simulink model "main_simplify"  (R2022a)
settings: Solver=ode4  StartTime=0.0  StopTime=1000  FixedStep=0.1  RelTol=1e-3
undefined symbols (not defined in the file): X, Y, Z
libraries: nesl_utility x28, sm_lib x9, sharedtransform x1
(part 1 of 2)
settings Model: Creator=sakur  LastModifiedBy=sakur

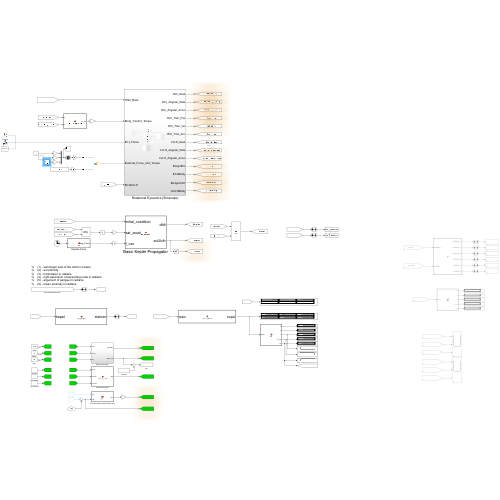
[thumbnail: Simulink's stored preview of the top-level diagram]
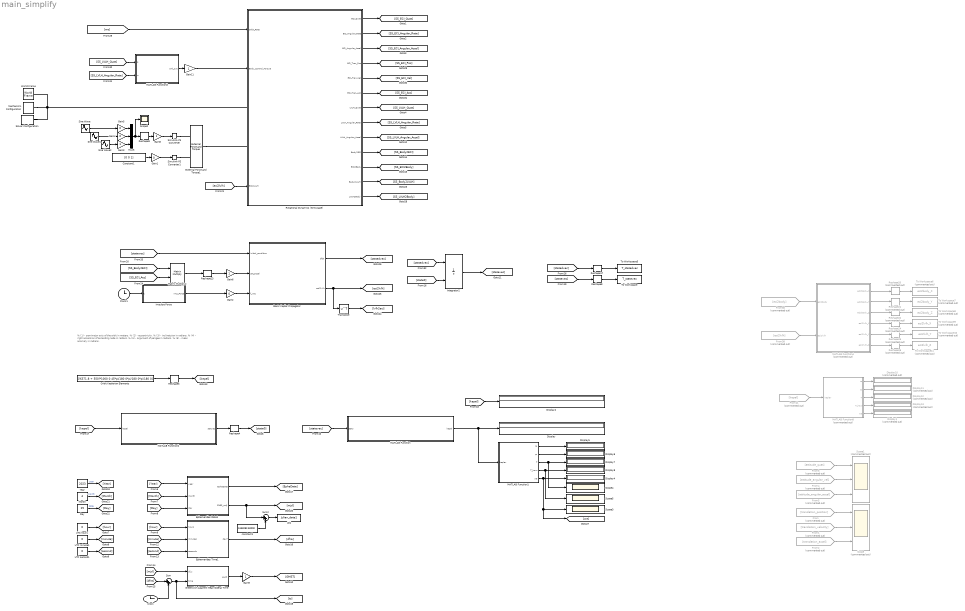
== system main_simplify ==
  note: %		(1) - semimajor axis of the orbit in meters.
      | %		(2) - eccentricity.
      | %		(3) - inclinatsion in radians.
      | %		(4) - right ascension of ascending node in radians.
      | %		(5) - argument of perigee in radians.
      | %		(6) - mean anomaly in radians.
  Basic Kepler Propagator : MATLAB Function  TreatAsAtomicUnit=on
  Clock : Clock
  Clock1 : Clock
  Constant1 : Constant  Value=[0 0 1]
  Day : Constant  Value=25
  Display{,2,4..8} (7 alike) : Display
  Display{1,10..13} (5 alike) : Display  Commented=on
  Ephemerides Date1 : Subsystem
  Ephemerides Time1 : MATLAB Function  TreatAsAtomicUnit=on
  External Force and Torque1 : sm_lib/Forces and Torques/External Force and Torque  ForceResolutionFrame=AttachedFrame  EnableForceX=off  EnableForceY=off  EnableForceZ=off  EnableForce=on  TorqueResolutionFrame=AttachedFrame  EnableTorqueX=off  EnableTorqueY=off  EnableTorqueZ=off  EnableTorque=on
  From : From  Commented=on  GotoTag=translation_position
  From1 : From  Commented=on  GotoTag=translation_velocity
  From11 : From  Commented=on  GotoTag=kepel
  From2 : From  Commented=on  GotoTag=translation_accel
  From3 : From  Commented=on  GotoTag=attitude_quat
  From36 : From  Commented=on  GotoTag=eci2body
  From38 : From  Commented=on  GotoTag=eci2lvlh
  From4 : From  Commented=on  GotoTag=attitude_angular_vel
  From5 : From  Commented=on  GotoTag=attitude_angular_accel
  Gain{1..2,4..5} (4 alike) : Gain  Gain=0
  Gain{3,6,8..9,11} (5 alike) : Gain
  Greenwich Aparent Mean Sideral Time : MATLAB Function  TreatAsAtomicUnit=on
  Impulse Force : MATLAB Function  TreatAsAtomicUnit=on
  Integrator2 : Integrator  InitialConditionSource=external  InitialCondition=[-7000 0 0 0 -9.175045 0 5233.5]'
  JD1 : ToWorkspace  VariableName=Julian_date1  SampleTime=-1
  MATLAB Function : MATLAB Function  TreatAsAtomicUnit=on
  MATLAB Function1 : MATLAB Function  TreatAsAtomicUnit=on
  MATLAB Function2 : MATLAB Function  TreatAsAtomicUnit=on
  MATLAB Function3 : MATLAB Function  TreatAsAtomicUnit=on
  MATLAB Function4 : MATLAB Function  Commented=on  TreatAsAtomicUnit=on
  MATLAB Function8 : MATLAB Function  Commented=on  TreatAsAtomicUnit=on
  Matrix Multiply2 : Product  Multiplication=Matrix(*)
  Mechanism Configuration : sm_lib/Utilities/Mechanism Configuration  UniformGravity=None  GravityVector=[0 0 -9.80665]  GravityUnits=m/s^2  LinearizationDelta=0.001  JointModeTransitionNonlinearIterations=2
  Month : Constant  Value=4
  Mux5 : Mux  Inputs=3
  Orbit Keplerian Elements : Constant  Value=[(6371.8 + 550)*1000 0 45*pi/180 0*pi/180 0*pi/180 0]
  Reshape{3..4,8,17} (4 alike) : Reshape  OutputDimensionality=Row vector (2-D)
  Reshape{20..22,24..26} (6 alike) : Reshape  Commented=on  OutputDimensionality=Row vector (2-D)
  Reshape23 : Reshape  OutputDimensionality=Customize  OutputDimensions=[3,1]
  Reshape9 : Reshape  OutputDimensionality=Column vector (2-D)
  Rotational Dynamics (Simscape) : Subsystem
      settings: PortSchema="{\"entries\":[{\"content\":{\"sides\":[{\"content\":{\"connectorIds\":[\"In1\",\"In2\",\"LConn1\",\"LConn2\",\"In3\"]},\"type\":\"ConnectorPlacement.EquallySpacedRectSide\",\"uuid\":\"81c45185-2b66-4f6c-94eb-3cfd86780641\"},{\"content\":{\"connectorIds\":[\"Out1\",\"Out2\",\"Out3\",\"Out4\",\"Out5\",\"Out6\",\"Out7\",\"Out8\",\"Out9\",\"Out10\",\"Out11\",\"Out12\",\"Out13\"],\"side\":\"RIGHT\"},\"type\":\"ConnectorPlacement.EquallySpacedRectSide\",\"uuid\":\"1106ea16-9c7f-47ad-94d6-2ae2f4fd049a\"},{\"content\":{\"connectorIds\":[],\"side\":\"TOP\"},\"type\":\"ConnectorPlacement.EquallySpacedRectSide\",\"uuid\":\"80c62f24-87e6-45ac-a7a8-c289464b6430\"}]},\"type\":\"ConnectorPlacement.EquallySpacedConnector\",\"uuid\":\"d3715883-22cc-4ca4-b826-d669ea23df66\"}],\"packageUris\":[\"http://schema.mathworks.com/mf0/Connector/R2020b\"],\"version\":\"1.0\"}"
  Scope : Scope  Commented=on  NumInputPorts=3
  Scope1 : Scope  Commented=on  NumInputPorts=3
  Scope{2..5} (4 alike) : Scope
  Simulink-PS Converter : nesl_utility/Simulink-PS Converter  PhysicalDomain=network_engine_domain  SubClassName=ps_input  LeftPortType=input  RightPortType=output  PseudoPeriodic=off  Frequencies=[]  NoiseDistribution=none  NoiseParameters=[]  Unit=1  AffineConversion=off  FilteringAndDerivatives=provide  SimscapeFilterOrder=1  InputFilterTimeConstant=0.001  UdotUserProvided=0
      settings: SourceProductBaseCode=SS,PW,VE
  Simulink-PS Converter1 : nesl_utility/Simulink-PS Converter  PhysicalDomain=network_engine_domain  SubClassName=ps_input  LeftPortType=input  RightPortType=output  PseudoPeriodic=off  Frequencies=[]  NoiseDistribution=none  NoiseParameters=[]  Unit=1  AffineConversion=off  FilteringAndDerivatives=provide  SimscapeFilterOrder=1  InputFilterTimeConstant=0.001  UdotUserProvided=0
      settings: SourceProductBaseCode=SS,PW,VE
  Sine Wave : Sin  Amplitude=0  Bias=10  SampleTime=0
  Sine Wave1 : Sin  Amplitude=0  Bias=10  SampleTime=0
  Sine Wave2 : Sin  Amplitude=0.0001  Frequency=0.01  SampleTime=0
  Solver Configuration : nesl_utility/Solver Configuration  PhysicalDomain=network_engine_domain  SubClassName=solver  LeftPortType=input  RightPortType=generic  Tones=[]  Harmonics=[]  SimulateNoise=off  Profile=off  UseLocalSampling=off  EnableSwitchedLinearOptims=on  FrequencyDomain=off  UseCCode=off  RelTol=0.001  AbsTol=0.001  MinStep=1e-09  ToWorkspace=off  RevertToSquareIcSolve=off  NumHomotopyIterations=100  PhasorMode=off  PhasorModeNumHarmonics=1  IndexReductionMethod=DerivativeReplacement  DoDC=off  ResidualTolerance=1e-09  UseLocalSolver=off  LocalSolverChoice=NE_BACKWARD_EULER_ADVANCER  LocalSolverSampleTime=0.001  DoFixedCost=off  MaxNonlinIter=3  MaxModeIter=2  ComputeImpulses=off  ImpulseIterations=2  LinearAlgebra=auto  LinearAlgebraNumThread=0  EquationFormulation=NE_TIME_EF  DelaysMemoryBudget=1024  AutomaticFiltering=on  FilteringTimeConstant=0.001  PartitionStorageMethod=AS_NEEDED  PartitionMemoryBudget=1024  PartitionMethod=ROBUST
      settings: SourceProductBaseCode=SS,PW,VE
  Sum : Sum  Inputs=|++
  Sum2 : Sum  Inputs=|++
  To Workspace : ToWorkspace  VariableName=T_statevec  SampleTime=-1
      settings: Save2DSignal=2-D array (concatenate along first dimension)
  To Workspace10 : ToWorkspace  Commented=on  VariableName=eci2lvlh_Y  SampleTime=-1
      settings: Save2DSignal=2-D array (concatenate along first dimension)
  To Workspace11 : ToWorkspace  Commented=on  VariableName=eci2lvlh_Z  SampleTime=-1
      settings: Save2DSignal=2-D array (concatenate along first dimension)
  To Workspace5 : ToWorkspace  VariableName=T_statedvec  SampleTime=-1
      settings: Save2DSignal=2-D array (concatenate along first dimension)
  To Workspace6 : ToWorkspace  Commented=on  VariableName=eci2body_X  SampleTime=-1
      settings: Save2DSignal=2-D array (concatenate along first dimension)
  To Workspace7 : ToWorkspace  Commented=on  VariableName=eci2body_Y  SampleTime=-1
      settings: Save2DSignal=2-D array (concatenate along first dimension)
  To Workspace8 : ToWorkspace  Commented=on  VariableName=eci2body_Z  SampleTime=-1
      settings: Save2DSignal=2-D array (concatenate along first dimension)
  To Workspace9 : ToWorkspace  Commented=on  VariableName=eci2lvlh_X  SampleTime=-1
      settings: Save2DSignal=2-D array (concatenate along first dimension)
  Transpose : Math  Operator=transpose
  UTC hour1 : Constant  Value=0
  UTC minute1 : Constant  Value=0
  UTC second1 : Constant  Value=0
  World Frame : sm_lib/Frames and Transforms/World Frame
  Year : Constant  Value=2023
  constant1 : Constant  Value=2433282.50000
  wires:
  Reshape17/1 -> To Workspace5/1
  MATLAB Function1/4(T_hour) -> Scope5/1, Display8/1
  MATLAB Function1/3(T) -> Scope4/1, Display7/1
  Gain8/1 -> Simulink-PS Converter/1
  Transpose/1 -> [lvlh2eci]
  MATLAB Function4/5(eci2lvlh_Y) -> Reshape25/1
  [statedvec] -> Integrator2/1
  MATLAB Function4/3(eci2body_Z) -> Reshape22/1
  From5/1 -> Scope1/3
  From38/1 -> MATLAB Function4/2(eci2lvlh)
  Reshape22/1 -> To Workspace8/1
  MATLAB Function1/5(we) -> [we], Scope3/1, Display4/1
  [SS_LVLH_Angular_Rate] -> MATLAB Function3/2(w)
  UTC hour1/1 -> [hour]
  MATLAB Function8/1(ra) -> Display10/1
  MATLAB Function4/4(eci2lvlh_X) -> Reshape24/1
  Reshape23/1 -> Gain6/1
  Matrix Multiply2/1 -> Reshape23/1
  [Year] -> Ephemerides Date1/1(year)
  MATLAB Function4/2(eci2body_Y) -> Reshape21/1
  From1/1 -> Scope/2
  Reshape26/1 -> To Workspace11/1
  [SS_ECI_Acc] -> Matrix Multiply2/2
  [SS_Body2ECI] -> Matrix Multiply2/1
  MATLAB Function3/1(cntl_out) -> Gain11/1
  Ephemerides Time1/1(dayf) -> [dfra]
  MATLAB Function4/1(eci2body_X) -> Reshape20/1
  Clock1/1 -> Impulse Force/1(t)
  Mux5/1 -> Scope2/1, Reshape9/1
  Gain1/1 -> Simulink-PS Converter1/1
  Reshape21/1 -> To Workspace7/1
  Day/1 -> [Day]  "date"
  Gain2/1 -> Basic Kepler Propagator/3(f_vec)
  MATLAB Function/1(kepel) -> Display/1, MATLAB Function1/1(kepler)
  [SS_LVLH_Quat] -> MATLAB Function3/1(q)
  MATLAB Function8/5(we) -> Display1/1
  Reshape24/1 -> To Workspace9/1
  MATLAB Function1/1(ra) -> Display5/1
  [statevec] -> Basic Kepler Propagator/1(initial_condition)
  Reshape3/1 -> [kepel]
  [kepel] -> MATLAB Function2/1(kepel)
  From2/1 -> Scope/3
  From11/1 -> MATLAB Function8/1(kepler)
  [dfra] -> Sum/1
  Orbit Keplerian Elements/1 -> Reshape3/1
  Reshape20/1 -> To Workspace6/1
  MATLAB Function8/4(T_hour) -> Display13/1
  Greenwich Aparent Mean Sideral Time/1(gwst) -> Gain9/1
  Year/1 -> [Year]  "year"
  Ephemerides Date1/2(CNES_mdj) -> Sum2/1, [mjd]
  From4/1 -> Scope1/2
  From3/1 -> Scope1/1
  UTC second1/1 -> [second]
  Constant1/1 -> Gain1/1
  [minute] -> Ephemerides Time1/2(minutes)
  Gain5/1 -> Mux5/1
  Basic Kepler Propagator/1(dfdt) -> [statedvec]
  constant1/1 -> Sum2/2
  Integrator2/1 -> [statevec]
  [state0] -> Integrator2/2
  MATLAB Function8/3(T) -> Display12/1
  From36/1 -> MATLAB Function4/1(eci2body)
  Sine Wave2/1 -> Gain3/1
  Impulse Force/1(Imp_Force) -> Gain2/1
  Clock/1 -> Sum/2
  [statedvec] -> Reshape17/1
  [Day] -> Ephemerides Date1/3(day)
  Gain4/1 -> Mux5/2
  Reshape8/1 -> To Workspace/1
  MATLAB Function4/6(eci2lvlh_Z) -> Reshape26/1
  Sum2/1 -> JD1/1
  Sum/1 -> Greenwich Aparent Mean Sideral Time/2(time), [ts]
  From/1 -> Scope/1
  Ephemerides Date1/1(EpheDate) -> [EpheDate]
  Gain3/1 -> Mux5/3
  [second] -> Ephemerides Time1/3(seconds)
  Sine Wave1/1 -> Gain4/1
  [hour] -> Ephemerides Time1/1(hours)
  Sine Wave/1 -> Gain5/1
  MATLAB Function2/1(statvec) -> Reshape4/1
  Reshape25/1 -> To Workspace10/1
  [Month] -> Ephemerides Date1/2(month)
  [statevec] -> MATLAB Function/1(statv)
  Reshape9/1 -> Gain8/1
  Basic Kepler Propagator/2(eci2lvlh) -> Transpose/1, [eci2lvlh]
  Reshape4/1 -> [state0]
  [kepel] -> Display2/1
  MATLAB Function1/2(rp) -> Display6/1
  MATLAB Function8/2(rp) -> Display11/1
  Gain9/1 -> [GMST]
  Month/1 -> [Month]  "month"
  Gain6/1 -> Basic Kepler Propagator/2(sat_accel)
  [mjd] -> Greenwich Aparent Mean Sideral Time/1(diju)
  [statevec] -> Reshape8/1
  UTC minute1/1 -> [minute]
  [we] -> Rotational Dynamics (Simscape)/1(Orbit_Rate)
  Gain11/1 -> Rotational Dynamics (Simscape)/2(Body_Control_Torque)
  [eci2lvlh] -> Rotational Dynamics (Simscape)/3(ECI2LVLH)
  Rotational Dynamics (Simscape)/1(ECI_Quat) -> [SS_ECI_Quat]
  Rotational Dynamics (Simscape)/2(ECI_Angular_Rate) -> [SS_ECI_Angular_Rate]
  Rotational Dynamics (Simscape)/3(ECI_Angular_Accel) -> [SS_ECI_Angular_Accel]
  Rotational Dynamics (Simscape)/7(LVLH_Quat) -> [SS_LVLH_Quat]
  Rotational Dynamics (Simscape)/8(LVLH_Angular_Rate) -> [SS_LVLH_Angular_Rate]
  Rotational Dynamics (Simscape)/9(LVLH_Angular_Accel) -> [SS_LVLH_Angular_Accel]
  Rotational Dynamics (Simscape)/10(Body2ECI) -> [SS_Body2ECI]
  Rotational Dynamics (Simscape)/11(ECI2Body) -> [SS_ECI2Body]
  Rotational Dynamics (Simscape)/12(Body2LVLH) -> [SS_Body2LVLH]
  Rotational Dynamics (Simscape)/13(LVLH2Body) -> [SS_LVLH2Body]
  Rotational Dynamics (Simscape)/4(ECI_Tran_Pos) -> [SS_ECI_Pos]
  Rotational Dynamics (Simscape)/5(ECI_Tran_Vel) -> [SS_ECI_Vel]
  Rotational Dynamics (Simscape)/6(ECI_Tran_Acc) -> [SS_ECI_Acc]
  connections:
  Simulink-PS Converter1/RConn1 -- External Force and Torque1/LConn2
  Simulink-PS Converter/RConn1 -- External Force and Torque1/LConn1
  Mechanism Configuration/RConn1 -- Solver Configuration/RConn1 -- Rotational Dynamics (Simscape)/LConn1 -- World Frame/RConn1
  External Force and Torque1/RConn1 -- Rotational Dynamics (Simscape)/LConn2

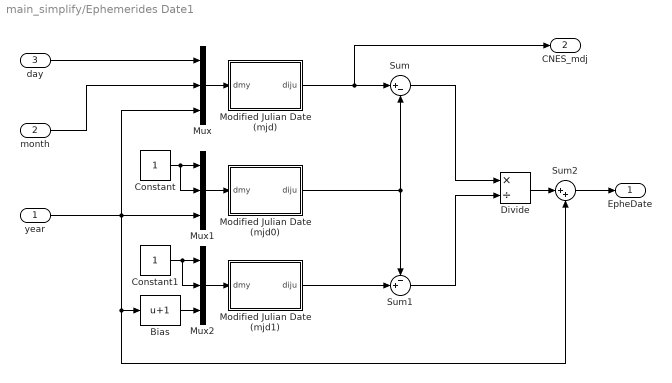
== system main_simplify/Ephemerides Date1 ==
  year : Inport
  month : Inport  Port=2
  day : Inport  Port=3
  Bias : Bias  Bias=1  SaturateOnIntegerOverflow=off
  Constant : Constant
  Constant1 : Constant
  Divide : Product  Inputs=*/
  Modified Julian Date (mjd) : MATLAB Function  TreatAsAtomicUnit=on
  Modified Julian Date (mjd0) : MATLAB Function  TreatAsAtomicUnit=on
  Modified Julian Date (mjd1) : MATLAB Function  TreatAsAtomicUnit=on
  Mux : Mux  Inputs=3
  Mux1 : Mux  Inputs=3
  Mux2 : Mux  Inputs=3
  Sum : Sum  Inputs=|+-
  Sum1 : Sum  Inputs=-+|
  Sum2 : Sum  Inputs=|++
  EpheDate : Outport
  CNES_mdj : Outport  Port=2
  wires:
  Sum1/1 -> Divide/2
  Modified Julian Date (mjd1)/1(diju) -> Sum1/2
  month/1 -> Mux/2
  year/1 -> Mux1/3, Mux/3, Bias/1, Sum2/2
  Mux1/1 -> Modified Julian Date (mjd0)/1(dmy)
  day/1 -> Mux/1
  Mux/1 -> Modified Julian Date (mjd)/1(dmy)
  Mux2/1 -> Modified Julian Date (mjd1)/1(dmy)
  Bias/1 -> Mux2/3
  Modified Julian Date (mjd)/1(diju) -> CNES_mdj/1, Sum/1
  Constant1/1 -> Mux2/2, Mux2/1
  Sum/1 -> Divide/1
  Constant/1 -> Mux1/2, Mux1/1
  Modified Julian Date (mjd0)/1(diju) -> Sum1/1, Sum/2
  Divide/1 -> Sum2/1
  Sum2/1 -> EpheDate/1

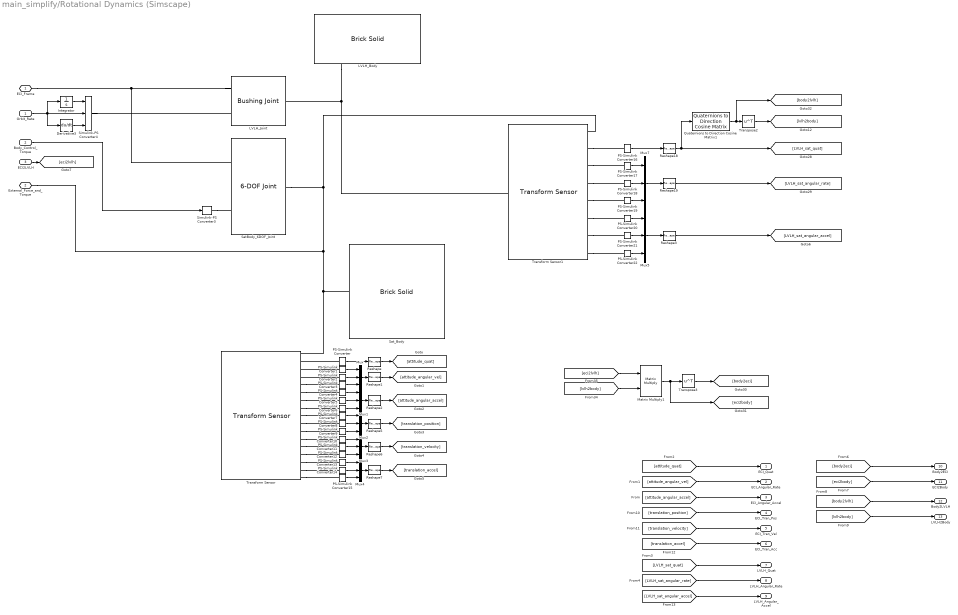
== system main_simplify/Rotational Dynamics (Simscape) ==
  Orbit_Rate : Inport
  Body_Control_Torque : Inport  Port=2
  ECI2LVLH : Inport  Port=3
  Derivative3 : Derivative
  Integrator : Integrator
  LVLH_Body : sm_lib/Body Elements/Brick Solid  GraphicAmbientColor=[0.15 0.15 0.15 1.0]  BasedOnType=Mass  BrickDimensions=[1 1 1]  BrickDimensionUnits=m  CenterOfMass=[0 0 0]  CenterOfMassUnits=m  GraphicDiffuseColor=[0.0 1.0 1.0]  Density=1000  DensityUnits=kg/m^3  DoExposeReferenceFrame=on  GraphicEmissiveColor=[0.0 0.0 0.0 1.0]  ExportEntireGeometry=off  SerializedFrames=<Frames><Frame><Id>Frame1</Id><Value><Name>CoM_F</Name><Origin><Source>CenterOfMassFrame</Source><FeatureName></FeatureName></Origin><PrimaryAxis><DefinedDirection>+Z</DefinedDirection><Source>ReferenceFrame</Source><SourceDirection>+Z</SourceDirection><FeatureName></FeatureName></PrimaryAxis><SecondaryAxis><DefinedDirection>+X</DefinedDirection><Source>ReferenceFrame</Source><SourceDirection>+X</SourceDirection><FeatureName></FeatureName></SecondaryAxis></Value></Frame><Frame><Id>Frame2</Id><Value><Name>LVLH_F</Name><Origin><Source>CenterOfMassFrame</Source><FeatureName></FeatureName></Origin><PrimaryAxis><DefinedDirection>+Z</DefinedDirection><Source>ReferenceFrame</Source><SourceDirection>+Z</SourceDirection><FeatureName></FeatureName></PrimaryAxis><SecondaryAxis><DefinedDirection>+X</DefinedDirection><Source>ReferenceFrame</Source><SourceDirection>+X</SourceDirection><FeatureName></FeatureName></SecondaryAxis></Value></Frame></Frames>  MarkerShape=Sphere  MarkerSize=10  GraphicType=FromGeometry  InertiaType=CalculateFromGeometry  Mass=0.000001  MassUnits=kg  MomentsOfInertia=[1 1 1]  MomentsOfInertiaUnits=kg*m^2  GraphicOpacity=0  ProductsOfInertia=[0 0 0]  ProductsOfInertiaUnits=kg*m^2  GraphicShininess=75  GraphicSpecularColor=[0.5 0.5 0.5 1.0]  GraphicVisPropType=SimpleVisualProperties
  LVLH_Joint : sm_lib/Joints/Bushing Joint  JointMode=Normal  SenseConstraintForce=off  SenseConstraintForceX=off  SenseConstraintForceY=off  SenseConstraintForceZ=off  SenseConstraintTorque=off  SenseConstraintTorqueX=off  SenseConstraintTorqueY=off  SenseConstraintTorqueZ=off  SenseTotalForce=off  SenseTotalForceX=off  SenseTotalForceY=off  SenseTotalForceZ=off  SenseTotalTorque=off  SenseTotalTorqueX=off  SenseTotalTorqueY=off  SenseTotalTorqueZ=off  CompositeWrenchDir=FollowerOnBase  CompositeWrenchFrame=BaseFrame  PxEquilibriumPosition=0  PxEquilibriumPositionUnits=m  PxSpringStiffness=0  PxSpringStiffnessUnits=N/m  PxDampingCoefficient=0  PxDampingCoefficientUnits=N/(m/s)  PxTorqueActuationMode=NoTorque  PxMotionActuationMode=ComputedMotion  PxSensePosition=off  PxSenseVelocity=off  PxSenseAcceleration=off  PxSenseTorqueForce=off  PxSenseLowerLimitTorqueForce=off  PxSenseUpperLimitTorqueForce=off  PxLowerLimitSpecify=off  PxLowerLimitBound=-1  PxLowerLimitBoundUnits=m  PxLowerLimitStiffness=1e6  PxLowerLimitStiffnessUnits=N/m  PxLowerLimitDamping=1e3  PxLowerLimitDampingUnits=N/(m/s)  PxLowerLimitTransitionRegionWidth=1e-4  PxLowerLimitTransitionRegionWidthUnits=m  PxUpperLimitSpecify=off  PxUpperLimitBound=1  PxUpperLimitBoundUnits=m  PxUpperLimitStiffness=1e6  PxUpperLimitStiffnessUnits=N/m  PxUpperLimitDamping=1e3  PxUpperLimitDampingUnits=N/(m/s)  PxUpperLimitTransitionRegionWidth=1e-4  PxUpperLimitTransitionRegionWidthUnits=m  PxPositionTargetSpecify=off  PxPositionTargetPriority=High  PxPositionTargetValue=0  PxPositionTargetValueUnits=m  PxVelocityTargetSpecify=off  PxVelocityTargetPriority=High  PxVelocityTargetValue=0  PxVelocityTargetValueUnits=m/s  PyEquilibriumPosition=0  PyEquilibriumPositionUnits=m  PySpringStiffness=0  PySpringStiffnessUnits=N/m  PyDampingCoefficient=0  PyDampingCoefficientUnits=N/(m/s)  PyTorqueActuationMode=NoTorque  PyMotionActuationMode=ComputedMotion  PySensePosition=off  PySenseVelocity=off  PySenseAcceleration=off  PySenseTorqueForce=off  PySenseLowerLimitTorqueForce=off  PySenseUpperLimitTorqueForce=off  PyLowerLimitSpecify=off  PyLowerLimitBound=-1  PyLowerLimitBoundUnits=m  PyLowerLimitStiffness=1e6  PyLowerLimitStiffnessUnits=N/m  PyLowerLimitDamping=1e3  PyLowerLimitDampingUnits=N/(m/s)  PyLowerLimitTransitionRegionWidth=1e-4  PyLowerLimitTransitionRegionWidthUnits=m  PyUpperLimitSpecify=off  PyUpperLimitBound=1  PyUpperLimitBoundUnits=m  PyUpperLimitStiffness=1e6  PyUpperLimitStiffnessUnits=N/m  PyUpperLimitDamping=1e3  PyUpperLimitDampingUnits=N/(m/s)  PyUpperLimitTransitionRegionWidth=1e-4  PyUpperLimitTransitionRegionWidthUnits=m  PyPositionTargetSpecify=off  PyPositionTargetPriority=High  PyPositionTargetValue=0  PyPositionTargetValueUnits=m  PyVelocityTargetSpecify=off  PyVelocityTargetPriority=High  PyVelocityTargetValue=0  PyVelocityTargetValueUnits=m/s  PzEquilibriumPosition=0  PzEquilibriumPositionUnits=m  PzSpringStiffness=0  PzSpringStiffnessUnits=N/m  PzDampingCoefficient=0  PzDampingCoefficientUnits=N/(m/s)  PzTorqueActuationMode=NoTorque  PzMotionActuationMode=ComputedMotion  PzSensePosition=off  PzSenseVelocity=off  PzSenseAcceleration=off  PzSenseTorqueForce=off  PzSenseLowerLimitTorqueForce=off  PzSenseUpperLimitTorqueForce=off  PzLowerLimitSpecify=off  PzLowerLimitBound=-1  PzLowerLimitBoundUnits=m  PzLowerLimitStiffness=1e6  PzLowerLimitStiffnessUnits=N/m  PzLowerLimitDamping=1e3  PzLowerLimitDampingUnits=N/(m/s)  PzLowerLimitTransitionRegionWidth=1e-4  PzLowerLimitTransitionRegionWidthUnits=m  PzUpperLimitSpecify=off  PzUpperLimitBound=1  PzUpperLimitBoundUnits=m  PzUpperLimitStiffness=1e6  PzUpperLimitStiffnessUnits=N/m  PzUpperLimitDamping=1e3  PzUpperLimitDampingUnits=N/(m/s)  PzUpperLimitTransitionRegionWidth=1e-4  PzUpperLimitTransitionRegionWidthUnits=m  PzPositionTargetSpecify=off  PzPositionTargetPriority=High  PzPositionTargetValue=0  PzPositionTargetValueUnits=m  PzVelocityTargetSpecify=off  PzVelocityTargetPriority=High  PzVelocityTargetValue=0  PzVelocityTargetValueUnits=m/s  RxEquilibriumPosition=0  RxEquilibriumPositionUnits=deg  RxSpringStiffness=0  RxSpringStiffnessUnits=N*m/deg  RxDampingCoefficient=0  RxDampingCoefficientUnits=N*m/(deg/s)  RxTorqueActuationMode=NoTorque  RxMotionActuationMode=ComputedMotion  RxSensePosition=off  RxSenseVelocity=off  RxSenseAcceleration=off  RxSenseTorqueForce=off  RxSenseLowerLimitTorqueForce=off  RxSenseUpperLimitTorqueForce=off  RxLowerLimitSpecify=off  RxLowerLimitBound=-90  RxLowerLimitBoundUnits=deg  RxLowerLimitStiffness=1e4  RxLowerLimitStiffnessUnits=N*m/deg  RxLowerLimitDamping=10  RxLowerLimitDampingUnits=N*m/(deg/s)  RxLowerLimitTransitionRegionWidth=0.1  RxLowerLimitTransitionRegionWidthUnits=deg  RxUpperLimitSpecify=off  RxUpperLimitBound=90  RxUpperLimitBoundUnits=deg  RxUpperLimitStiffness=1e4  RxUpperLimitStiffnessUnits=N*m/deg  RxUpperLimitDamping=10  RxUpperLimitDampingUnits=N*m/(deg/s)  RxUpperLimitTransitionRegionWidth=0.1  RxUpperLimitTransitionRegionWidthUnits=deg  RxPositionTargetSpecify=off  RxPositionTargetPriority=High  RxPositionTargetValue=0  RxPositionTargetValueUnits=deg  RxVelocityTargetSpecify=off  RxVelocityTargetPriority=High  RxVelocityTargetValue=0  RxVelocityTargetValueUnits=deg/s  RyEquilibriumPosition=0  RyEquilibriumPositionUnits=deg  RySpringStiffness=0  RySpringStiffnessUnits=N*m/deg  RyDampingCoefficient=0  RyDampingCoefficientUnits=N*m/(deg/s)  RyTorqueActuationMode=ComputedTorque  RyMotionActuationMode=InputMotion  RySensePosition=off  RySenseVelocity=off  RySenseAcceleration=off  RySenseTorqueForce=off  RySenseLowerLimitTorqueForce=off  RySenseUpperLimitTorqueForce=off  RyLowerLimitSpecify=off  RyLowerLimitBound=-90  RyLowerLimitBoundUnits=deg  RyLowerLimitStiffness=1e4  RyLowerLimitStiffnessUnits=N*m/deg  RyLowerLimitDamping=10  RyLowerLimitDampingUnits=N*m/(deg/s)  RyLowerLimitTransitionRegionWidth=0.1  RyLowerLimitTransitionRegionWidthUnits=deg  RyUpperLimitSpecify=off  RyUpperLimitBound=90  RyUpperLimitBoundUnits=deg  RyUpperLimitStiffness=1e4  RyUpperLimitStiffnessUnits=N*m/deg  RyUpperLimitDamping=10  RyUpperLimitDampingUnits=N*m/(deg/s)  RyUpperLimitTransitionRegionWidth=0.1  RyUpperLimitTransitionRegionWidthUnits=deg  RyPositionTargetSpecify=off  RyPositionTargetPriority=High  RyPositionTargetValue=0  RyPositionTargetValueUnits=deg  RyVelocityTargetSpecify=off  RyVelocityTargetPriority=High  RyVelocityTargetValue=0  RyVelocityTargetValueUnits=deg/s  RzEquilibriumPosition=0  RzEquilibriumPositionUnits=deg  RzSpringStiffness=0  RzSpringStiffnessUnits=N*m/deg  RzDampingCoefficient=0  RzDampingCoefficientUnits=N*m/(deg/s)  RzTorqueActuationMode=NoTorque  RzMotionActuationMode=ComputedMotion  RzSensePosition=off  RzSenseVelocity=off  RzSenseAcceleration=off  RzSenseTorqueForce=off  RzSenseLowerLimitTorqueForce=off  RzSenseUpperLimitTorqueForce=off  RzLowerLimitSpecify=off  RzLowerLimitBound=-90  RzLowerLimitBoundUnits=deg  RzLowerLimitStiffness=1e4  RzLowerLimitStiffnessUnits=N*m/deg  RzLowerLimitDamping=10  RzLowerLimitDampingUnits=N*m/(deg/s)  RzLowerLimitTransitionRegionWidth=0.1  RzLowerLimitTransitionRegionWidthUnits=deg  RzUpperLimitSpecify=off  RzUpperLimitBound=90  RzUpperLimitBoundUnits=deg  RzUpperLimitStiffness=1e4  RzUpperLimitStiffnessUnits=N*m/deg  RzUpperLimitDamping=10  RzUpperLimitDampingUnits=N*m/(deg/s)  RzUpperLimitTransitionRegionWidth=0.1  RzUpperLimitTransitionRegionWidthUnits=deg  RzPositionTargetSpecify=off  RzPositionTargetPriority=High  RzPositionTargetValue=0  RzPositionTargetValueUnits=deg  RzVelocityTargetSpecify=off  RzVelocityTargetPriority=High  RzVelocityTargetValue=0  RzVelocityTargetValueUnits=deg/s
  Matrix Multiply1 : Product  Multiplication=Matrix(*)
  Mux{,1..5,7} (7 alike) : Mux  Inputs=3
  PS-Simulink Converter{,1..22} (23 alike) : nesl_utility/PS-Simulink Converter  PhysicalDomain=network_engine_domain  SubClassName=ps_output  LeftPortType=input  RightPortType=output  PseudoPeriodic=off  Frequencies=[]  VectorFormat=inherit  Unit=inherit  AffineConversion=off
      settings: SourceProductBaseCode=SS,PW,VE
  Quaternions to Direction Cosine Matrix1 : sharedtransform/Quaternions to  Direction Cosine Matrix  aMode=aMode
      settings: SourceProductBaseCode=AE,PW,DR,MT,VE
  Reshape{,1..3,5..7,18..19} (9 alike) : Reshape  OutputDimensionality=Column vector (2-D)
  SatBody_6DOF_Joint : sm_lib/Joints/6-DOF Joint  JointMode=Normal  SenseConstraintForce=off  SenseConstraintForceX=off  SenseConstraintForceY=off  SenseConstraintForceZ=off  SenseConstraintTorque=off  SenseConstraintTorqueX=off  SenseConstraintTorqueY=off  SenseConstraintTorqueZ=off  SenseTotalForce=off  SenseTotalForceX=off  SenseTotalForceY=off  SenseTotalForceZ=off  SenseTotalTorque=off  SenseTotalTorqueX=off  SenseTotalTorqueY=off  SenseTotalTorqueZ=off  CompositeWrenchDir=FollowerOnBase  CompositeWrenchFrame=BaseFrame  PxEquilibriumPosition=0  PxEquilibriumPositionUnits=m  PxSpringStiffness=0  PxSpringStiffnessUnits=N/m  PxDampingCoefficient=0  PxDampingCoefficientUnits=N/(m/s)  PxTorqueActuationMode=NoTorque  PxMotionActuationMode=ComputedMotion  PxSensePosition=off  PxSenseVelocity=off  PxSenseAcceleration=off  PxSenseTorqueForce=off  PxSenseLowerLimitTorqueForce=off  PxSenseUpperLimitTorqueForce=off  PxLowerLimitSpecify=off  PxLowerLimitBound=-1  PxLowerLimitBoundUnits=m  PxLowerLimitStiffness=1e6  PxLowerLimitStiffnessUnits=N/m  PxLowerLimitDamping=1e3  PxLowerLimitDampingUnits=N/(m/s)  PxLowerLimitTransitionRegionWidth=1e-4  PxLowerLimitTransitionRegionWidthUnits=m  PxUpperLimitSpecify=off  PxUpperLimitBound=1  PxUpperLimitBoundUnits=m  PxUpperLimitStiffness=1e6  PxUpperLimitStiffnessUnits=N/m  PxUpperLimitDamping=1e3  PxUpperLimitDampingUnits=N/(m/s)  PxUpperLimitTransitionRegionWidth=1e-4  PxUpperLimitTransitionRegionWidthUnits=m  PxPositionTargetSpecify=off  PxPositionTargetPriority=High  PxPositionTargetValue=0  PxPositionTargetValueUnits=m  PxVelocityTargetSpecify=off  PxVelocityTargetPriority=High  PxVelocityTargetValue=0  PxVelocityTargetValueUnits=m/s  PyEquilibriumPosition=0  PyEquilibriumPositionUnits=m  PySpringStiffness=0  PySpringStiffnessUnits=N/m  PyDampingCoefficient=0  PyDampingCoefficientUnits=N/(m/s)  PyTorqueActuationMode=NoTorque  PyMotionActuationMode=ComputedMotion  PySensePosition=off  PySenseVelocity=off  PySenseAcceleration=off  PySenseTorqueForce=off  PySenseLowerLimitTorqueForce=off  PySenseUpperLimitTorqueForce=off  PyLowerLimitSpecify=off  PyLowerLimitBound=-1  PyLowerLimitBoundUnits=m  PyLowerLimitStiffness=1e6  PyLowerLimitStiffnessUnits=N/m  PyLowerLimitDamping=1e3  PyLowerLimitDampingUnits=N/(m/s)  PyLowerLimitTransitionRegionWidth=1e-4  PyLowerLimitTransitionRegionWidthUnits=m  PyUpperLimitSpecify=off  PyUpperLimitBound=1  PyUpperLimitBoundUnits=m  PyUpperLimitStiffness=1e6  PyUpperLimitStiffnessUnits=N/m  PyUpperLimitDamping=1e3  PyUpperLimitDampingUnits=N/(m/s)  PyUpperLimitTransitionRegionWidth=1e-4  PyUpperLimitTransitionRegionWidthUnits=m  PyPositionTargetSpecify=off  PyPositionTargetPriority=High  PyPositionTargetValue=0  PyPositionTargetValueUnits=m  PyVelocityTargetSpecify=off  PyVelocityTargetPriority=High  PyVelocityTargetValue=0  PyVelocityTargetValueUnits=m/s  PzEquilibriumPosition=0  PzEquilibriumPositionUnits=m  PzSpringStiffness=0  PzSpringStiffnessUnits=N/m  PzDampingCoefficient=0  PzDampingCoefficientUnits=N/(m/s)  PzTorqueActuationMode=NoTorque  PzMotionActuationMode=ComputedMotion  PzSensePosition=off  PzSenseVelocity=off  PzSenseAcceleration=off  PzSenseTorqueForce=off  PzSenseLowerLimitTorqueForce=off  PzSenseUpperLimitTorqueForce=off  PzLowerLimitSpecify=off  PzLowerLimitBound=-1  PzLowerLimitBoundUnits=m  PzLowerLimitStiffness=1e6  PzLowerLimitStiffnessUnits=N/m  PzLowerLimitDamping=1e3  PzLowerLimitDampingUnits=N/(m/s)  PzLowerLimitTransitionRegionWidth=1e-4  PzLowerLimitTransitionRegionWidthUnits=m  PzUpperLimitSpecify=off  PzUpperLimitBound=1  PzUpperLimitBoundUnits=m  PzUpperLimitStiffness=1e6  PzUpperLimitStiffnessUnits=N/m  PzUpperLimitDamping=1e3  PzUpperLimitDampingUnits=N/(m/s)  PzUpperLimitTransitionRegionWidth=1e-4  PzUpperLimitTransitionRegionWidthUnits=m  PzPositionTargetSpecify=off  PzPositionTargetPriority=High  PzPositionTargetValue=0  PzPositionTargetValueUnits=m  PzVelocityTargetSpecify=off  PzVelocityTargetPriority=High  PzVelocityTargetValue=0  PzVelocityTargetValueUnits=m/s  SphDefPosRotationMethod=None  SphDefPosRotationAngleUnits=deg  SphDefPosRotationStandardAxis=+Z  SphDefPosRotationAngle=0.0  SphDefPosRotationArbitraryAxis=[0 0 1]  SphDefPosFollAlignAxisA=+X  SphDefPosBaseAlignAxisA=+Y  SphDefPosFollAlignAxisB=+Y  SphDefPosBaseAlignAxisB=+Z  SphDefPosRotationSequenceAxes=FollowerAxes  SphDefPosRotationSequence=XYX  SphDefPosRotationSequenceAngles=[0 0 0]  SphDefPosRotationSequenceAnglesUnits=deg  SphDefPosRotationMatrix=[1 0 0; 0 1 0; 0 0 1]  SphEqPosRotationMethod=None  SphEqPosRotationAngleUnits=deg  SphEqPosRotationStandardAxis=+Z  SphEqPosRotationAngle=0.0  SphEqPosRotationArbitraryAxis=[0 0 1]  SphEqPosFollAlignAxisA=+X  SphEqPosBaseAlignAxisA=+Y  SphEqPosFollAlignAxisB=+Y  SphEqPosBaseAlignAxisB=+Z  SphEqPosRotationSequenceAxes=FollowerAxes  SphEqPosRotationSequence=XYX  SphEqPosRotationSequenceAngles=[0 0 0]  SphEqPosRotationSequenceAnglesUnits=deg  SphEqPosRotationMatrix=[1 0 0; 0 1 0; 0 0 1]  SphSpringStiffness=0  SphSpringStiffnessUnits=N*m/deg  SphDampingCoefficient=0  SphDampingCoefficientUnits=N*m/(deg/s)  SphActuateTorqueX=off  SphActuateTorqueY=off  SphActuateTorqueZ=off  SphActuateTorque=on  SphTorqueActuationMode=InputTorque  SphMotionActuationMode=ComputedMotion  SphActuationFrame=FollowerFrame  SphSensePosition=off  SphSenseVelocityX=off  SphSenseVelocityY=off  SphSenseVelocityZ=off  SphSenseVelocity=off  SphSenseAccelerationX=off  SphSenseAccelerationY=off  SphSenseAccelerationZ=off  SphSenseAcceleration=off  SphSenseTorqueX=off  SphSenseTorqueY=off  SphSenseTorqueZ=off  SphSenseTorqueForce=off  SphSenseLowerLimitTorqueMag=off  SphSenseUpperLimitTorqueMag=off  SphSensingFrame=BaseFrame  SphLowerLimitSpecify=off  SphLowerLimitBound=15  SphLowerLimitBoundUnits=deg  SphLowerLimitStiffness=1e4  SphLowerLimitStiffnessUnits=N*m/deg  SphLowerLimitDamping=10  SphLowerLimitDampingUnits=N*m/(deg/s)  SphLowerLimitTransitionRegionWidth=0.1  SphLowerLimitTransitionRegionWidthUnits=deg  SphUpperLimitSpecify=off  SphUpperLimitBound=45  SphUpperLimitBoundUnits=deg  SphUpperLimitStiffness=1e4  SphUpperLimitStiffnessUnits=N*m/deg  SphUpperLimitDamping=10  SphUpperLimitDampingUnits=N*m/(deg/s)  SphUpperLimitTransitionRegionWidth=0.1  SphUpperLimitTransitionRegionWidthUnits=deg  SphPositionTargetRotationMethod=RotationSequence  SphPositionTargetRotationAngleUnits=deg  SphPositionTargetRotationStandardAxis=+Z  SphPositionTargetRotationAngle=0.0  SphPositionTargetRotationArbitraryAxis=[0 0 1]  SphPositionTargetFollAlignAxisA=+X  SphPositionTargetBaseAlignAxisA=+Y  SphPositionTargetFollAlignAxisB=+Y  SphPositionTargetBaseAlignAxisB=+Z  SphPositionTargetRotationSequenceAxes=FollowerAxes  SphPositionTargetRotationSequence=ZYX  SphPositionTargetRotationSequenceAngles=[0 0 0]  SphPositionTargetRotationSequenceAnglesUnits=deg  SphPositionTargetRotationMatrix=[1 0 0; 0 1 0; 0 0 1]  SphPositionTargetSpecify=on  SphPositionTargetPriority=High  SphVelocityTargetValue=[0 0 0]  SphVelocityTargetValueUnits=deg/s  SphVelocityTargetSpecify=off  SphVelocityTargetPriority=High  SphVelocityTargetInFollowerFrame=on
  Sat_Body : sm_lib/Body Elements/Brick Solid  GraphicAmbientColor=[0.15 0.15 0.15 1.0]  BasedOnType=Mass  BrickDimensions=[1 1 1]  BrickDimensionUnits=m  CenterOfMass=[0 0 0]  CenterOfMassUnits=m  GraphicDiffuseColor=[0.0 1.0 1.0]  Density=1000  DensityUnits=kg/m^3  DoExposeReferenceFrame=on  GraphicEmissiveColor=[0.0 0.0 0.0 1.0]  ExportEntireGeometry=off  SerializedFrames=<Frames><Frame><Id>Frame1</Id><Value><Name>CoM_F</Name><Origin><Source>CenterOfMassFrame</Source><FeatureName></FeatureName></Origin><PrimaryAxis><DefinedDirection>+Z</DefinedDirection><Source>ReferenceFrame</Source><SourceDirection>+Z</SourceDirection><FeatureName></FeatureName></PrimaryAxis><SecondaryAxis><DefinedDirection>+X</DefinedDirection><Source>ReferenceFrame</Source><SourceDirection>+X</SourceDirection><FeatureName></FeatureName></SecondaryAxis></Value></Frame></Frames>  MarkerShape=Sphere  MarkerSize=10  GraphicType=FromGeometry  InertiaType=CalculateFromGeometry  Mass=10  MassUnits=kg  MomentsOfInertia=[1 1 1]  MomentsOfInertiaUnits=kg*m^2  GraphicOpacity=1.0  ProductsOfInertia=[0 0 0]  ProductsOfInertiaUnits=kg*m^2  GraphicShininess=75  GraphicSpecularColor=[0.5 0.5 0.5 1.0]  GraphicVisPropType=SimpleVisualProperties
  Simulink-PS Converter3 : nesl_utility/Simulink-PS Converter  PhysicalDomain=network_engine_domain  SubClassName=ps_input  LeftPortType=input  RightPortType=output  PseudoPeriodic=off  Frequencies=[]  NoiseDistribution=none  NoiseParameters=[]  Unit=1  AffineConversion=off  FilteringAndDerivatives=provide  SimscapeFilterOrder=1  InputFilterTimeConstant=0.001  UdotUserProvided=0
      settings: SourceProductBaseCode=SS,PW,VE
  Simulink-PS Converter4 : nesl_utility/Simulink-PS Converter  PhysicalDomain=network_engine_domain  SubClassName=ps_input  LeftPortType=input  RightPortType=output  PseudoPeriodic=off  Frequencies=[]  NoiseDistribution=none  NoiseParameters=[]  Unit=1  AffineConversion=off  FilteringAndDerivatives=provide  SimscapeFilterOrder=1  InputFilterTimeConstant=0.001  UdotUserProvided=2
      settings: SourceProductBaseCode=SS,PW,VE
  Transform Sensor : sm_lib/Frames and Transforms/Transform Sensor  MeasurementFrame=World  SenseAngle=off  SenseAxis=off  SenseAngle1=off  SenseAngle2=off  SenseAngle3=off  SenseQ=on  SenseR=off  SenseOmegaX=on  SenseOmegaY=on  SenseOmegaZ=on  SenseOmega1=off  SenseOmega2=off  SenseOmega3=off  SenseQDot=off  SenseRDot=off  SenseAlphaX=on  SenseAlphaY=on  SenseAlphaZ=on  SenseAlpha1=off  SenseAlpha2=off  SenseAlpha3=off  SenseQDDot=off  SenseRDDot=off  SenseX=on  SenseY=on  SenseZ=on  SenseRad=off  SenseAzim=off  SenseDist=off  SenseInc=off  SenseXDot=on  SenseYDot=on  SenseZDot=on  SenseRadDot=off  SenseAzimDot=off  SenseDistDot=off  SenseIncDot=off  SenseXDDot=on  SenseYDDot=on  SenseZDDot=on  SenseRadDDot=off  SenseAzimDDot=off  SenseDistDDot=off  SenseIncDDot=off
  Transform Sensor1 : sm_lib/Frames and Transforms/Transform Sensor  MeasurementFrame=Follower  SenseAngle=off  SenseAxis=off  SenseAngle1=off  SenseAngle2=off  SenseAngle3=off  SenseQ=on  SenseR=off  SenseOmegaX=on  SenseOmegaY=on  SenseOmegaZ=on  SenseOmega1=off  SenseOmega2=off  SenseOmega3=off  SenseQDot=off  SenseRDot=off  SenseAlphaX=on  SenseAlphaY=on  SenseAlphaZ=on  SenseAlpha1=off  SenseAlpha2=off  SenseAlpha3=off  SenseQDDot=off  SenseRDDot=off  SenseX=off  SenseY=off  SenseZ=off  SenseRad=off  SenseAzim=off  SenseDist=off  SenseInc=off  SenseXDot=off  SenseYDot=off  SenseZDot=off  SenseRadDot=off  SenseAzimDot=off  SenseDistDot=off  SenseIncDot=off  SenseXDDot=off  SenseYDDot=off  SenseZDDot=off  SenseRadDDot=off  SenseAzimDDot=off  SenseDistDDot=off  SenseIncDDot=off
  Transpose2 : Math  Operator=transpose
  Transpose3 : Math  Operator=transpose
  ECI_Frame : PMIOPort  Side=Left
  External_Force_and_Torque : PMIOPort  Port=2  Side=Left
  ECI_Quat : Outport
  ECI_Angular_Rate : Outport  Port=2
  ECI_Angular_Accel : Outport  Port=3
  ECI_Tran_Pos : Outport  Port=4
  ECI_Tran_Vel : Outport  Port=5
  ECI_Tran_Acc : Outport  Port=6
  LVLH_Quat : Outport  Port=7
  LVLH_Angular_Rate : Outport  Port=8
  LVLH_Angular_Accel : Outport  Port=9
  Body2ECI : Outport  Port=10
  ECI2Body : Outport  Port=11
  Body2LVLH : Outport  Port=12
  LVLH2Body : Outport  Port=13
  wires:
  PS-Simulink Converter2/1 -> Mux/2
  Reshape5/1 -> [translation_position]
  Reshape7/1 -> [translation_accel]
  Matrix Multiply1/1 -> Transpose3/1, [eci2body]
  Mux3/1 -> Reshape6/1
  PS-Simulink Converter19/1 -> Mux7/3
  Reshape6/1 -> [translation_velocity]
  PS-Simulink Converter12/1 -> Mux3/3
  Reshape1/1 -> [attitude_angular_vel]
  PS-Simulink Converter4/1 -> Mux1/1
  PS-Simulink Converter8/1 -> Mux2/2
  PS-Simulink Converter13/1 -> Mux4/1
  PS-Simulink Converter15/1 -> Mux4/3
  PS-Simulink Converter6/1 -> Mux1/3
  Quaternions to Direction Cosine Matrix1/1 -> [body2lvlh], Transpose2/1
  Body_Control_Torque/1 -> Simulink-PS Converter3/1
  PS-Simulink Converter5/1 -> Mux1/2
  Transpose2/1 -> [lvlh2body]
  PS-Simulink Converter9/1 -> Mux2/3
  PS-Simulink Converter17/1 -> Mux7/1
  Reshape19/1 -> [LVLH_sat_angular_rate]
  Derivative3/1 -> Simulink-PS Converter4/3
  PS-Simulink Converter11/1 -> Mux3/2
  PS-Simulink Converter3/1 -> Mux/3
  Mux7/1 -> Reshape19/1
  [eci2lvlh] -> Matrix Multiply1/1
  PS-Simulink Converter16/1 -> Reshape18/1
  Reshape18/1 -> [LVLH_sat_quat], Quaternions to Direction Cosine Matrix1/1
  [lvlh2body] -> Matrix Multiply1/2
  PS-Simulink Converter18/1 -> Mux7/2
  Reshape2/1 -> [attitude_angular_accel]
  Transpose3/1 -> [body2eci]
  Mux4/1 -> Reshape7/1
  Mux1/1 -> Reshape2/1
  PS-Simulink Converter1/1 -> Mux/1
  PS-Simulink Converter7/1 -> Mux2/1
  PS-Simulink Converter/1 -> Reshape/1
  Orbit_Rate/1 -> Derivative3/1, Integrator/1, Simulink-PS Converter4/2
  PS-Simulink Converter10/1 -> Mux3/1
  PS-Simulink Converter14/1 -> Mux4/2
  Integrator/1 -> Simulink-PS Converter4/1
  Mux/1 -> Reshape1/1
  Reshape/1 -> [attitude_quat]
  Mux2/1 -> Reshape5/1
  [attitude_angular_accel] -> ECI_Angular_Accel/1
  [attitude_angular_vel] -> ECI_Angular_Rate/1
  [attitude_quat] -> ECI_Quat/1
  [LVLH_sat_quat] -> LVLH_Quat/1
  [LVLH_sat_angular_accel] -> LVLH_Angular_Accel/1
  [LVLH_sat_angular_rate] -> LVLH_Angular_Rate/1
  Mux5/1 -> Reshape3/1
  PS-Simulink Converter20/1 -> Mux5/1
  PS-Simulink Converter21/1 -> Mux5/2
  Reshape3/1 -> [LVLH_sat_angular_accel]
  PS-Simulink Converter22/1 -> Mux5/3
  [body2eci] -> Body2ECI/1
  [eci2body] -> ECI2Body/1
  [lvlh2body] -> LVLH2Body/1
  [body2lvlh] -> Body2LVLH/1
  ECI2LVLH/1 -> [eci2lvlh]
  [translation_position] -> ECI_Tran_Pos/1
  [translation_velocity] -> ECI_Tran_Vel/1
  [translation_accel] -> ECI_Tran_Acc/1
  connections:
  Transform Sensor/RConn14 -- PS-Simulink Converter12/LConn1
  PS-Simulink Converter/LConn1 -- Transform Sensor/RConn2
  Transform Sensor/RConn16 -- PS-Simulink Converter14/LConn1
  LVLH_Body/LConn1 -- LVLH_Joint/RConn1 -- Transform Sensor1/LConn1
  Transform Sensor/RConn7 -- PS-Simulink Converter5/LConn1
  Transform Sensor/RConn13 -- PS-Simulink Converter11/LConn1
  LVLH_Joint/LConn1 -- ECI_Frame/RConn1 -- SatBody_6DOF_Joint/LConn1
  Simulink-PS Converter3/RConn1 -- SatBody_6DOF_Joint/LConn2
  Transform Sensor1/RConn4 -- PS-Simulink Converter18/LConn1
  SatBody_6DOF_Joint/RConn1 -- Transform Sensor/RConn1 -- Sat_Body/LConn1 -- External_Force_and_Torque/RConn1 -- Transform Sensor1/RConn1
  Transform Sensor/RConn12 -- PS-Simulink Converter10/LConn1
  Transform Sensor/RConn11 -- PS-Simulink Converter9/LConn1
  Transform Sensor1/RConn2 -- PS-Simulink Converter16/LConn1
  Transform Sensor/RConn9 -- PS-Simulink Converter7/LConn1
  Transform Sensor1/RConn3 -- PS-Simulink Converter17/LConn1
  Transform Sensor/RConn8 -- PS-Simulink Converter6/LConn1
  Transform Sensor/RConn10 -- PS-Simulink Converter8/LConn1
  Simulink-PS Converter4/RConn1 -- LVLH_Joint/LConn2
  Transform Sensor/RConn5 -- PS-Simulink Converter3/LConn1
  Transform Sensor/RConn15 -- PS-Simulink Converter13/LConn1
  Transform Sensor/RConn17 -- PS-Simulink Converter15/LConn1
  Transform Sensor/RConn6 -- PS-Simulink Converter4/LConn1
  Transform Sensor1/RConn5 -- PS-Simulink Converter19/LConn1
  PS-Simulink Converter1/LConn1 -- Transform Sensor/RConn3
  PS-Simulink Converter2/LConn1 -- Transform Sensor/RConn4
  Transform Sensor1/RConn7 -- PS-Simulink Converter21/LConn1
  Transform Sensor1/RConn6 -- PS-Simulink Converter20/LConn1
  Transform Sensor1/RConn8 -- PS-Simulink Converter22/LConn1

== matlab function main_simplify/Ephemerides Date1/Modified Julian Date (mjd1) ==
  data: dmy input; diju output
function diju  =  djm (dmy)
% [diju] = djm (day, month, year)
%    The function djm furnishes the Modified Julian
%    Date with reference to the day, month and year,
%    at zero hours of the day.
% inputs:
%   dmy(1): day, day of the month
%   dmy(2): month, month of the year
%   dmy(3): year

% outputs:
%   diju
%       Modified Julian Date in days, referred to 1950.0. 
%
% Valdemir Carrara, Apr, 2003
%

diju = 367*dmy(3) + dmy(1) - 712269 + fix(275*dmy(2)/9)- fix(7*(dmy(3)+fix((dmy(2)+9)/12))/4);

== matlab function main_simplify/Ephemerides Time1 ==
  data: hours input; dayf output; minutes input; seconds input
function dayf  = time_to_dayf(hours, minutes, seconds)
% [dayf] = time_to_dayf (hours, minutes, seconds)
%    The function time_to_dayf returns with the day elapesed
%    time in seconds
% inputs:
%   hours     
%       day hour (integer).
%   minutes
%       minutes (integer).
%   seconds
%       seconds and fraction of second
% outputs:
%   dayf
%       Day elapsed time in seconds. 
%
% Valdemir Carrara, Feb, 2009
%

dayf = seconds + 60*(minutes + 60*hours);

== matlab function main_simplify/MATLAB Function8 ==
  data: kepler input; ra output; rp output; T output; T_hour output; we output
function [ra, rp, T, T_hour, we] = fcn(kepler)

u=3.9865*10^14;

a = kepler(1);
e = kepler(2);
% 

ra = a*(1+e);%장반경
rp = a*(1-e);%단반경

a = (ra+rp)/2;% semi-major axis

% a = (550 + 6371.8)*1000;

T = 2*pi*sqrt((a*a*a)/(u));

T_hour = T/3600;

we = 2*pi/T;
% we = 1.1207*0.001;

end

== matlab function main_simplify/MATLAB Function ==
  data: statv input; kepel output
function kepel  = statvec_kepel (statv)
% [kepel] = statvec_kepel (statv)
%
%	The function statvec_kepel transforms the state vector statv
%	into the corresponding keplerian elements in the
%	same reference system.
%
% Input:
%	statv
%		state vector in meters and meters/second.
%
% Output:
%	statvec_kepel
%		vector containing the keplerian elements:
%		(1) - semimajor axis of the orbit in meters.
%		(2) - eccentricity.
%		(3) - inclination in radians.
%		(4) - right ascension of ascending node in radians.
%		(5) - argument of perigee in radians.
%		(6) - mean anomaly in radians.
%
% Authors:
%	Helio K. Kuga
%    Valder M. Medeiros
%	Valdemir Carrara			february/80			version 1.0
%	Helio K. Kuga     			august/82           version 2.0
%	Ulisses T V Guedes 			december/95	 		version 2.1
%               - fix perigee procedure when orbit plane
%                  equal to equatorial plane
%	Valdemir Carrara 			july/05				(C version)
%   Valdemir Carrara            March/09        Matlab

EARTH_GRAVITY	= 3.9860064e+14;		% Earth's gravitational constant (m**3/s**2)

xp  = [statv(1) statv(2) statv(3)];
xv  = [statv(4) statv(5) statv(6)];
r      = sqrt(xp*xp');
vq     = xv*xv';
ainv   = 2.0/r - vq/EARTH_GRAVITY;

h      = cross(xp, xv);
hm     = sqrt(h*h');
an = [0 0 0];
if (hm < 1.e-10)
    disp (' *** Message from function statvec_kepel: *** ');
    disp (' There are no keplerian elements corresponding to this state vector');
    kepel = [0, 0, 0, 0, 0, 0];
else
    h      = h/hm;
    incl   = acos(h(3));
    raan   = atan2(h(1), -h(2));
    d      = xp*xv' / EARTH_GRAVITY;
    esene  = d * sqrt(EARTH_GRAVITY*ainv);
    ecose  = 1 - r*ainv;
    exc    = sqrt(esene*esene + ecose*ecose);
    E      = atan2(esene, ecose);
    mean   = mod (E - esene, 2*pi);
    if mean < 0
        mean = mean + 2*pi;
    end

    if exc < 1.e-10
        arpe = 0;
    else
        dp     = 1./r - ainv;
        ev     = dp*xp - d*xv;
        abev   = sqrt(ev*ev');
        ev     = ev/abev;
        an(1)  = cos(raan);
        an(2)  = sin(raan);
        an(3)  = 0;
        fi     = ev*cross(h, an)';
        arpe = acos(ev*an');
        if fi < 0
            arpe  =  -arpe + 2*pi;
        end
    end

    kepel = [1./ainv, exc, incl, raan, arpe, mean];
end

end

== matlab function main_simplify/Basic Kepler Propagator ==
  data: initial_condition input; sat_accel input; dfdt output; f_vec input; eci2lvlh output
function [dfdt, eci2lvlh]   = eq_propagate(initial_condition, sat_accel, f_vec)

u  = 3.9865*10^14;
Re = 6378137; % earth radius in m
sat_mass = 100;%[kg]

dfdt = zeros(size(initial_condition));

x  = initial_condition(1); % x
y  = initial_condition(2); % y
z  = initial_condition(3); % z
x1 = initial_condition(4); % vel_x
y1 = initial_condition(5); % vel_y
z1 = initial_condition(6); % vel_z

r=sqrt(x^2+y^2+z^2);

% % %   Keplar Motion Equatnion
% % %  => r_dd + u/(r^3)r_ = 0 => r_dd = -u/(r^3)r_
dfdt(1) = x1;% vel_x
dfdt(2) = y1;% vel_y
dfdt(3) = z1;% vel_z
dfdt(4) = -u*x/r^3 + sat_accel(1) + f_vec(1)/sat_mass;% accel_x
dfdt(5) = -u*y/r^3 + sat_accel(2) + f_vec(2)/sat_mass;% accel_y
dfdt(6) = -u*z/r^3 + sat_accel(3) + f_vec(3)/sat_mass;% accel_z

% % % % % % % % % % % % LVLH Frame % % % % % % % % % % % % % % % % % % % % % % % % % % % % % % % % % % % %
% x as the unit vector directed along the spacecraft position vector:
lvlh_z = -[x;y;z]./r; 
rcv    = cross([x;y;z],[x1;y1;z1]);
% z as the unit vector directed along the spacecraft's orbital angular momentum vector:
lvlh_y = rcv/norm(rcv);
% y as the unit vector that completes a right handed coordinate system:
lvlh_x = cross(lvlh_z, lvlh_y);

eci2lvlh = [lvlh_x, lvlh_y, lvlh_z];

end

== matlab function main_simplify/MATLAB Function2 ==
  data: kepel input; statvec output
function statvec  = kepel_statvec (kepel)
%  [statvec] = kepel_statvec (kepel)
%	The function kepel_statvec transforms the keplerian
%	elements kepel into the corresponding state vector in
%	the same reference system.
%
% Input:
%	kepel
% 		vector containing the keplerian elements:
%		(1) - semimajor axis of the orbit in meters.
%		(2) - eccentricity.
%		(3) - inclinatsion in radians.
%		(4) - right ascension of ascending node in radians.
%		(5) - argument of perigee in radians.
%		(6) - mean anomaly in radians.
% Output:
%	statvec
%  		state vector in meters and meters/second.
%
% Authors:
%	Helio K. Kuga;
%	Valder M. Medeiros;
%	Valdemir Carrara		february/80		version 1.0
%	Valdemir Carrara		july 2005		(C version)
%   Valdemir Carrara            March/09        Matlab

EARTH_GRAVITY	= 3.9860064e+14;		% Earth's gravitational constant (m**3/s**2)

a    = kepel(1);	% semi-major axis
exc  = kepel(2);	% eccentricity

c1   = sqrt(1. - exc*exc);

%     rotation matrix

orb2iner = rotmaz(-kepel(4))*rotmax(-kepel(3))*rotmaz(-kepel(5));

%     Kepler's equation

E    = kepler(kepel(6), exc);

sE   = sin(E);
cE   = cos(E);
c3   = sqrt(EARTH_GRAVITY/a)/(1. - exc*cE);

%     state vector

statvec = [[a*(cE - exc), a*c1*sE, 0]*orb2iner', [-c3*sE, c1*c3*cE, 0]*orb2iner'];

end

function [rot_mat] = rotmax (angle)
% [rot_mat] = rotmax (angle)
%   To obtain the rotation matrix around the X axis given the
%   rotation angle.
% inputs:
%   angle
%       rotation angle, in radians.
% outputs:
%   rot_mat
%       rotation matrix (3, 3)
%

% Valdemir Carrara, Sep, 1998

coan    =  cos(angle);
sian    =  sin(angle);

rot_mat =  [1, 0, 0; 0, coan, sian; 0, -sian, coan];

end

function [rot_mat] = rotmay (angle)
% [rot_mat] = rotmay (angle)
%   To obtain the rotation matrix around the Y axis given the
%   rotation angle.
% inputs:
%   angle
%       rotation angle, in radians.
% outputs:
%   rot_mat
%       rotation matrix (3, 3)
%

% Valdemir Carrara, Sep, 1998


coan    =  cos(angle);
sian    =  sin(angle);

rot_mat =  [coan, 0, -sian; 0, 1, 0; sian, 0, coan];

end

function [rot_mat] = rotmaz (angle)
% [rot_mat] = rotmaz (angle)
%   To obtain the rotation matrix around the Z axis given the
%   rotation angle.
% inputs:
%   angle
%       rotation angle, in radians.
% outputs:
%   rot_mat
%       rotation matrix (3, 3)
%

% Valdemir Carrara, Sep, 1998

coan    =  cos(angle);
sian    =  sin(angle);

rot_mat =  [coan, sian, 0; -sian, coan, 0; 0, 0, 1];
end

function [eccentric] = kepler (mean_anomaly, eccentricity)
% [eccentric] = kepler (mean_anomaly, eccentricity)
%	The subroutine kepler finds a solution to the
%	kepler's equation.
%
% Input:
%	mean_anomaly
%		mean anomaly in radians.
%	eccentricity
%		eccentricity.
%
% Output:
%	eccentric
%		eccentric anomaly in radians.
%
% Authors:
%	Valder M. de Medeiros		june/81		version 2.0
%	Valdemir Carrara			july 2005	(C version)
%   Valdemir Carrara            March/09        Matlab

exc2    = eccentricity*eccentricity;
am1     = mod (mean_anomaly, 2*pi);
am2     = am1 + am1;
am3     = am1 + am2;
shoot   = am1 + eccentricity*(1. - 0.125*exc2)*sin(am1) + ...
		0.5*exc2*(sin(am2) + 0.75*eccentricity*sin(am3));
shoot   = mod (shoot, 2*pi);

e1      = 1.0;
ic      = 0;

while ((abs(e1) > 1.e-12) && (ic <= 10)) 
	e1    = (shoot - am1 - eccentricity*sin(shoot)) / ...
			(1.0 - eccentricity*cos(shoot));
    shoot = shoot - e1;
    ic    = ic + 1;
end

if (ic >= 10)
    disp ('warning ** subroutine kepler did not converge in 10 iterations');
end

eccentric = shoot;


end

== matlab function main_simplify/MATLAB Function1 ==
  data: kepler input; ra output; rp output; T output; T_hour output; we output
function [ra, rp, T, T_hour, we] = fcn(kepler)

u=3.9865*10^14;

a = kepler(1);
e = kepler(2);
% 

ra = a*(1+e);%장반경
rp = a*(1-e);%단반경

a = (ra+rp)/2;% semi-major axis

% a = (550 + 6371.8)*1000;

T = 2*pi*sqrt((a*a*a)/(u));

T_hour = T/3600;

we = 2*pi/T;
% we = 1.1207*0.001;

end

== matlab function main_simplify/Impulse Force ==
  settings: updateMethod=DISCRETE
  data: Imp_Force output; t input
function Imp_Force  = fcn(t)

Imp_Force = [0 0 0]';

if ((t >= 1000) && (t <= 1050))
    Imp_Force =  [-10000 0 10000]';
elseif ((t >= 1100) && (t <= 1150))
    Imp_Force = -[-20000 0 10000]';
else
    Imp_Force = [0 0 0]';

end

end

== matlab function main_simplify/MATLAB Function3 ==
  data: q input; cntl_out output; w input
function cntl_out = LVLH_Attitude_Control(q, w)

qs = q(1);
qv = [q(2), q(3), q(4)]';
w  = [w(1), w(2), w(3)]';

K1 = diag([0.05 0.05 0.05]);
K2 = diag([0.4 0.4 0.4]);

cntl_out = K1*qv - K2*w;

end
